simulink model "FLCS"  (Simulink 6.0)
settings: Solver=FixedStepDiscrete  StartTime=0.0  StopTime=2  RelTol=1e-3
libraries: simulink x9
settings Model: Creator=valery  LastModifiedBy=root  ExtModeAutoUpdateStatusClock=off  ProdHWDeviceType=Motorola PowerPC
settings OptimizationCC: OptimizeModelRefInitCode=on  LifeSpan=1
settings HardwareCC: ProdEndianess=BigEndian  ProdHWDeviceType=Motorola PowerPC
settings RTWCC: SystemTargetFile=mpc555rt.tlc  TemplateMakefile=mpc555rt.tmf  Description=Embedded Target for Motorola MPC555 (real-time target)  ProcessScript=mpc555rt_make_rtw_hook
settings CodeAppCC: IgnoreCustomStorageClasses=off
settings STFCustomTargetCC: TargetFcnLib=diab_tfl_tmw.mat  GenFloatMathFcnCalls=ISO_C  ModelReferenceCompliant=off  CombineOutputUpdateFcns=on  ERTCustomFileBanners=on  SystemTargetFile=mpc555rt.tlc
settings ERTTargetCC: TargetFcnLib=diab_tfl_tmw.mat  GenFloatMathFcnCalls=ISO_C  ModelReferenceCompliant=off  SupportContinuousTime=on  SupportNonInlinedSFcns=on  InlinedParameterPlacement=NonHierarchical  RootIOFormat=Individual Arguments  ERTCustomFileTemplate=example_file_process.tlc  InitialValueSource=Model
settings CustomProperty: DataType=RTWOptions_EnumType__toolbox_rtw_targets_mpc555dk_mpc555dk_mpc555rt_MPC555_OPTIMIZATION_SWITCH  Value=speed
settings EnumStrPairs: String=speed

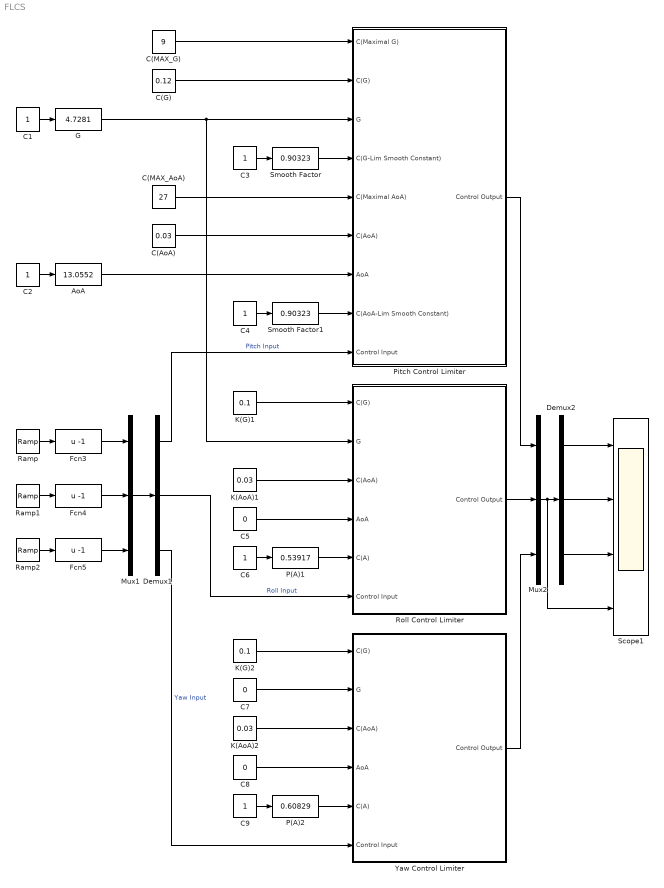
== system FLCS ==
  AoA : simulink/Math Operations/Slider Gain  low=1  gain=13.0552  high=25
  C(AoA) : Constant  Value=0.03
  C(G) : Constant  Value=0.12
  C(MAX_AoA) : Constant  Value=27
  C(MAX_G) : Constant  Value=9
  C{1..4,6,9} (6 alike) : Constant
  C5 : Constant  Value=0
  C7 : Constant  Value=0
  C8 : Constant  Value=0
  Demux1 : Demux  Outputs=3
  Demux2 : Demux  Outputs=3
  Fcn3 : Fcn  Expr=u -1
  Fcn4 : Fcn  Expr=u -1
  Fcn5 : Fcn  Expr=u -1
  G : simulink/Math Operations/Slider Gain  low=0  gain=4.7281  high=9
  K(AoA)1 : Constant  Value=0.03
  K(AoA)2 : Constant  Value=0.03
  K(G)1 : Constant  Value=0.1
  K(G)2 : Constant  Value=0.1
  Mux1 : Mux  Inputs=3
  Mux2 : Mux  Inputs=3
  P(A)1 : simulink/Math Operations/Slider Gain  low=0  gain=0.53917  high=1
  P(A)2 : simulink/Math Operations/Slider Gain  low=0  gain=0.60829  high=1
  Pitch Control Limiter : Subsystem
  Ramp : simulink/Sources/Ramp  slope=1  start=0  X0=0
  Ramp1 : simulink/Sources/Ramp  slope=1  start=0  X0=0
  Ramp2 : simulink/Sources/Ramp  slope=1  start=0  X0=0
  Roll Control Limiter : Subsystem
  Scope1 : Scope  NumInputPorts=4
      settings: YMin=-1.2~-1.2~-1.2~-1.1  YMax=1.2~1.2~1.2~1.1
  Smooth Factor : simulink/Math Operations/Slider Gain  low=0  gain=0.90323  high=1
  Smooth Factor1 : simulink/Math Operations/Slider Gain  low=0  gain=0.90323  high=1
  Yaw Control Limiter : Subsystem
  wires:
  Ramp/1 -> Fcn3/1
  Ramp1/1 -> Fcn4/1
  Ramp2/1 -> Fcn5/1
  Mux1/1 -> Demux1/1
  Fcn3/1 -> Mux1/1
  Fcn4/1 -> Mux1/2
  Fcn5/1 -> Mux1/3
  C1/1 -> G/1
  G/1 -> Pitch Control Limiter/3(G), Roll Control Limiter/2(G)
  C2/1 -> AoA/1
  C(G)/1 -> Pitch Control Limiter/2(C(G))
  Mux2/1 -> Demux2/1, Scope1/4
  Demux2/3 -> Scope1/3
  Demux2/2 -> Scope1/2
  Demux2/1 -> Scope1/1
  Demux1/1 -> Pitch Control Limiter/9(Control Input)  "Pitch Input"
  Pitch Control Limiter/1(Control Output) -> Mux2/1
  C3/1 -> Smooth Factor/1
  Smooth Factor/1 -> Pitch Control Limiter/4(C(G-Lim Smooth Constant))
  K(G)1/1 -> Roll Control Limiter/1(C(G))
  K(AoA)1/1 -> Roll Control Limiter/3(C(AoA))
  C6/1 -> P(A)1/1
  P(A)1/1 -> Roll Control Limiter/5(C(A))
  Roll Control Limiter/1(Control Output) -> Mux2/2
  Demux1/2 -> Roll Control Limiter/6(Control Input)  "Roll Input"
  C7/1 -> Yaw Control Limiter/2(G)
  C8/1 -> Yaw Control Limiter/4(AoA)
  K(G)2/1 -> Yaw Control Limiter/1(C(G))
  K(AoA)2/1 -> Yaw Control Limiter/3(C(AoA))
  C9/1 -> P(A)2/1
  P(A)2/1 -> Yaw Control Limiter/5(C(A))
  Yaw Control Limiter/1(Control Output) -> Mux2/3
  Demux1/3 -> Yaw Control Limiter/6(Control Input)  "Yaw Input"
  C5/1 -> Roll Control Limiter/4(AoA)
  C(MAX_G)/1 -> Pitch Control Limiter/1("C(Maximal G) ")
  AoA/1 -> Pitch Control Limiter/7(AoA)
  C4/1 -> Smooth Factor1/1
  Smooth Factor1/1 -> Pitch Control Limiter/8(C(AoA-Lim Smooth Constant))
  C(AoA)/1 -> Pitch Control Limiter/6(C(AoA))
  C(MAX_AoA)/1 -> Pitch Control Limiter/5(C(Maximal AoA))

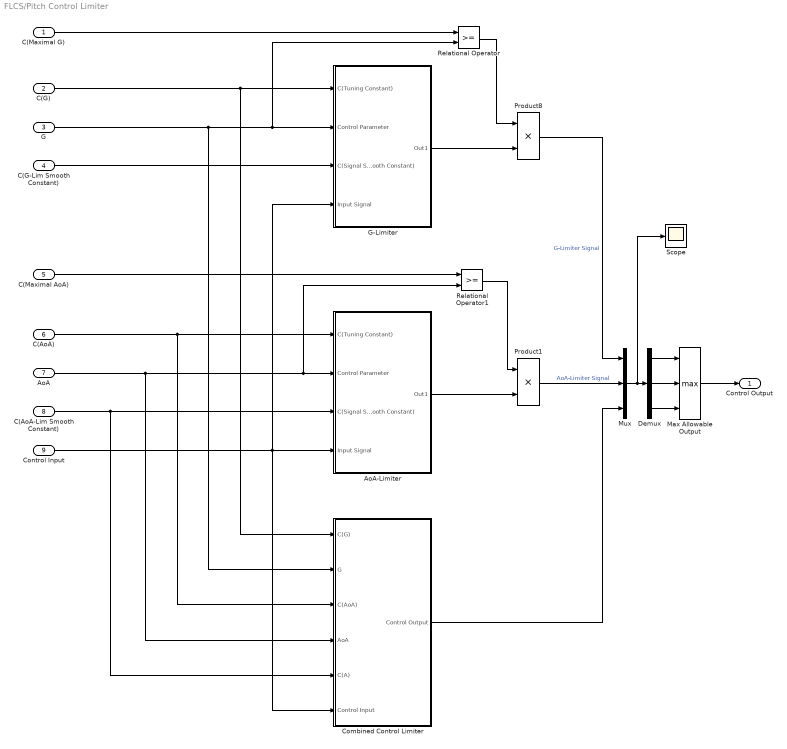
== system FLCS/Pitch Control Limiter ==
  "C(Maximal G) " : Inport  Port=1  LatchInput=off
  C(G) : Inport  Port=2  LatchInput=off
  G : Inport  Port=3  LatchInput=off
  C(G-Lim Smooth Constant) : Inport  Port=4  LatchInput=off
  C(Maximal AoA) : Inport  Port=5  LatchInput=off
  C(AoA) : Inport  Port=6  LatchInput=off
  AoA : Inport  Port=7  LatchInput=off
  C(AoA-Lim Smooth Constant) : Inport  Port=8  LatchInput=off
  Control Input : Inport  Port=9  LatchInput=off
  AoA-Limiter : Subsystem
  Combined Control Limiter : Subsystem
  Demux : Demux  Outputs=3
  G-Limiter : Subsystem
  Max Allowable Output : MinMax  Function=max  Inputs=3
  Mux : Mux  Inputs=3
  Product1 : Product  RndMeth=Zero
  Product8 : Product  RndMeth=Zero
  Relational Operator : RelationalOperator  LogicOutDataTypeMode=Boolean
  Relational Operator1 : RelationalOperator  LogicOutDataTypeMode=Boolean
  Scope : Scope
      settings: YMin=-1.1  YMax=1.1
  Control Output : Outport
  wires:
  "C(Maximal G) "/1 -> Relational Operator/1
  Relational Operator/1 -> Product8/1
  G-Limiter/1(Out1) -> Product8/2
  C(G)/1 -> G-Limiter/1(C(Tuning Constant)), Combined Control Limiter/1(C(G))
  G/1 -> G-Limiter/2(Control Parameter), Relational Operator/2, Combined Control Limiter/2(G)
  C(G-Lim Smooth Constant)/1 -> G-Limiter/3(C(Signal Smooth Constant))
  C(AoA)/1 -> AoA-Limiter/1(C(Tuning Constant)), Combined Control Limiter/3(C(AoA))
  C(AoA-Lim Smooth Constant)/1 -> AoA-Limiter/3(C(Signal Smooth Constant)), Combined Control Limiter/5(C(A))
  C(Maximal AoA)/1 -> Relational Operator1/1
  Relational Operator1/1 -> Product1/1
  AoA-Limiter/1(Out1) -> Product1/2
  Control Input/1 -> AoA-Limiter/4(Input Signal), G-Limiter/4(Input Signal), Combined Control Limiter/6(Control Input)
  Max Allowable Output/1 -> Control Output/1
  Product1/1 -> Mux/2  "AoA-Limiter Signal"
  Product8/1 -> Mux/1  "G-Limiter Signal"
  Combined Control Limiter/1(Control Output) -> Mux/3
  AoA/1 -> AoA-Limiter/2(Control Parameter), Relational Operator1/2, Combined Control Limiter/4(AoA)
  Mux/1 -> Demux/1, Scope/1
  Demux/1 -> Max Allowable Output/1
  Demux/2 -> Max Allowable Output/2
  Demux/3 -> Max Allowable Output/3

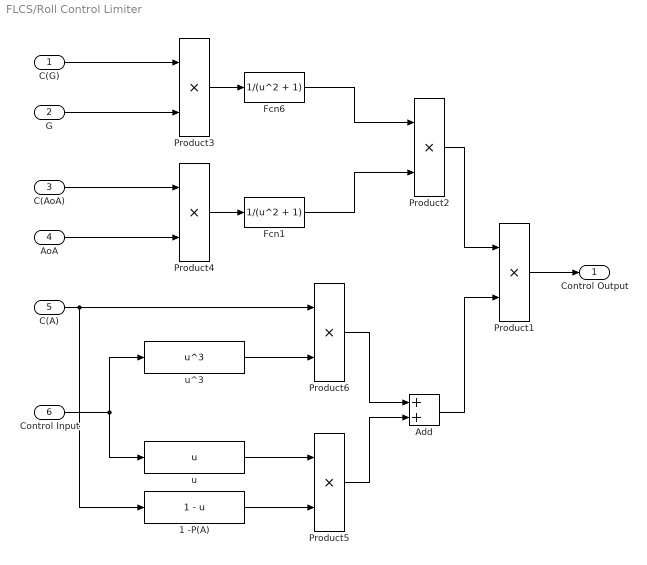
== system FLCS/Roll Control Limiter ==
  C(G) : Inport  Port=1  LatchInput=off
  G : Inport  Port=2  LatchInput=off
  C(AoA) : Inport  Port=3  LatchInput=off
  AoA : Inport  Port=4  LatchInput=off
  C(A) : Inport  Port=5  LatchInput=off
  Control Input : Inport  Port=6  LatchInput=off
  1 -P(A) : Fcn  Expr=1 - u
  Add : Sum  OutScaling=2^-10
  Fcn1 : Fcn  Expr=1/(u^2 + 1)
  Fcn6 : Fcn  Expr=1/(u^2 + 1)
  Product{1..6} (6 alike) : Product  RndMeth=Zero
  u : Fcn  Expr=u
  u^3 : Fcn  Expr=u^3
  Control Output : Outport
  wires:
  Product1/1 -> Control Output/1
  Control Input/1 -> u^3/1, u/1
  C(G)/1 -> Product3/1
  Product3/1 -> Fcn6/1
  Product4/1 -> Fcn1/1
  C(A)/1 -> 1 -P(A)/1, Product6/1
  u^3/1 -> Product6/2
  Product6/1 -> Add/1
  Product5/1 -> Add/2
  u/1 -> Product5/1
  1 -P(A)/1 -> Product5/2
  C(AoA)/1 -> Product4/1
  AoA/1 -> Product4/2
  G/1 -> Product3/2
  Fcn6/1 -> Product2/1
  Fcn1/1 -> Product2/2
  Add/1 -> Product1/2
  Product2/1 -> Product1/1

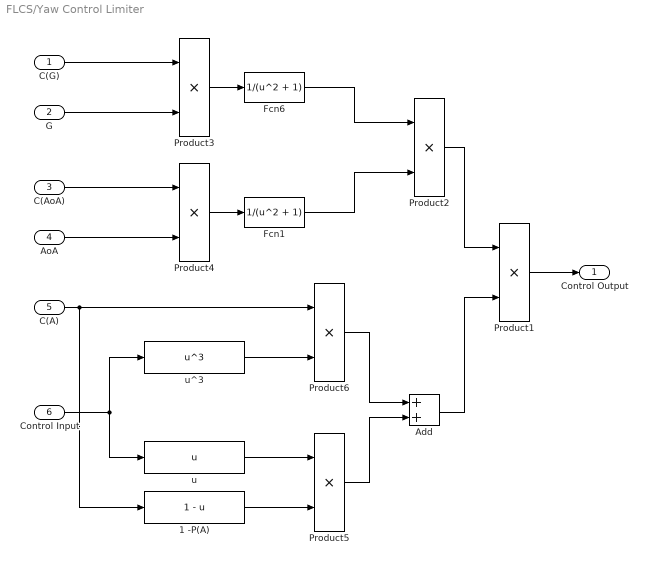
== system FLCS/Yaw Control Limiter ==
  C(G) : Inport  Port=1  LatchInput=off
  G : Inport  Port=2  LatchInput=off
  C(AoA) : Inport  Port=3  LatchInput=off
  AoA : Inport  Port=4  LatchInput=off
  C(A) : Inport  Port=5  LatchInput=off
  Control Input : Inport  Port=6  LatchInput=off
  1 -P(A) : Fcn  Expr=1 - u
  Add : Sum  OutScaling=2^-10
  Fcn1 : Fcn  Expr=1/(u^2 + 1)
  Fcn6 : Fcn  Expr=1/(u^2 + 1)
  Product{1..6} (6 alike) : Product  RndMeth=Zero
  u : Fcn  Expr=u
  u^3 : Fcn  Expr=u^3
  Control Output : Outport
  wires:
  Product1/1 -> Control Output/1
  Control Input/1 -> u^3/1, u/1
  C(G)/1 -> Product3/1
  Product3/1 -> Fcn6/1
  Product4/1 -> Fcn1/1
  C(A)/1 -> 1 -P(A)/1, Product6/1
  u^3/1 -> Product6/2
  Product6/1 -> Add/1
  Product5/1 -> Add/2
  u/1 -> Product5/1
  1 -P(A)/1 -> Product5/2
  C(AoA)/1 -> Product4/1
  AoA/1 -> Product4/2
  G/1 -> Product3/2
  Fcn6/1 -> Product2/1
  Fcn1/1 -> Product2/2
  Add/1 -> Product1/2
  Product2/1 -> Product1/1

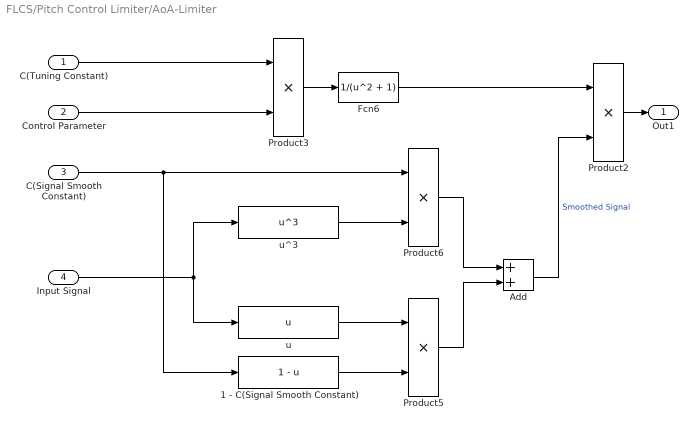
== system FLCS/Pitch Control Limiter/AoA-Limiter ==
  C(Tuning Constant) : Inport  Port=1  LatchInput=off
  Control Parameter : Inport  Port=2  LatchInput=off
  C(Signal Smooth Constant) : Inport  Port=3  LatchInput=off
  Input Signal : Inport  Port=4  LatchInput=off
  1 - C(Signal Smooth Constant) : Fcn  Expr=1 - u
  Add : Sum  OutScaling=2^-10
  Fcn6 : Fcn  Expr=1/(u^2 + 1)
  Product{2..3,5..6} (4 alike) : Product  RndMeth=Zero
  u : Fcn  Expr=u
  u^3 : Fcn  Expr=u^3
  Out1 : Outport
  wires:
  Input Signal/1 -> u/1, u^3/1
  C(Tuning Constant)/1 -> Product3/1
  Product3/1 -> Fcn6/1
  C(Signal Smooth Constant)/1 -> Product6/1, 1 - C(Signal Smooth Constant)/1
  u^3/1 -> Product6/2
  Product6/1 -> Add/1
  Product5/1 -> Add/2
  u/1 -> Product5/1
  1 - C(Signal Smooth Constant)/1 -> Product5/2
  Control Parameter/1 -> Product3/2
  Fcn6/1 -> Product2/1
  Add/1 -> Product2/2  "Smoothed Signal"
  Product2/1 -> Out1/1

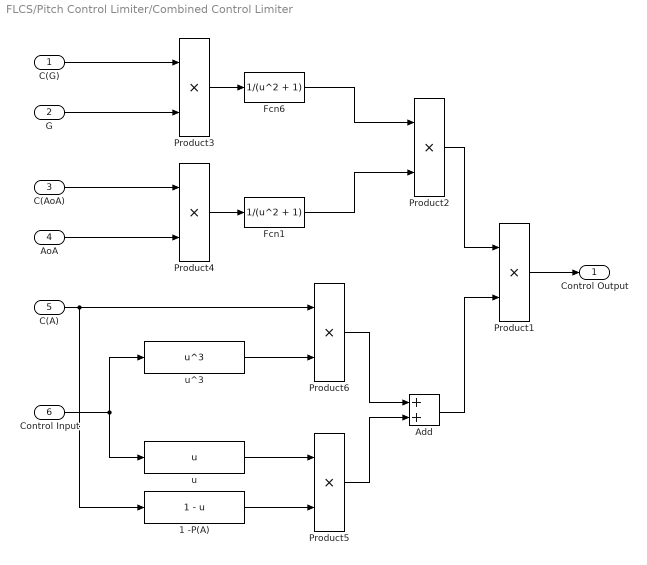
== system FLCS/Pitch Control Limiter/Combined Control Limiter ==
  C(G) : Inport  Port=1  LatchInput=off
  G : Inport  Port=2  LatchInput=off
  C(AoA) : Inport  Port=3  LatchInput=off
  AoA : Inport  Port=4  LatchInput=off
  C(A) : Inport  Port=5  LatchInput=off
  Control Input : Inport  Port=6  LatchInput=off
  1 -P(A) : Fcn  Expr=1 - u
  Add : Sum  OutScaling=2^-10
  Fcn1 : Fcn  Expr=1/(u^2 + 1)
  Fcn6 : Fcn  Expr=1/(u^2 + 1)
  Product{1..6} (6 alike) : Product  RndMeth=Zero
  u : Fcn  Expr=u
  u^3 : Fcn  Expr=u^3
  Control Output : Outport
  wires:
  Product1/1 -> Control Output/1
  Control Input/1 -> u^3/1, u/1
  C(G)/1 -> Product3/1
  Product3/1 -> Fcn6/1
  Product4/1 -> Fcn1/1
  C(A)/1 -> 1 -P(A)/1, Product6/1
  u^3/1 -> Product6/2
  Product6/1 -> Add/1
  Product5/1 -> Add/2
  u/1 -> Product5/1
  1 -P(A)/1 -> Product5/2
  C(AoA)/1 -> Product4/1
  AoA/1 -> Product4/2
  G/1 -> Product3/2
  Fcn6/1 -> Product2/1
  Fcn1/1 -> Product2/2
  Add/1 -> Product1/2
  Product2/1 -> Product1/1

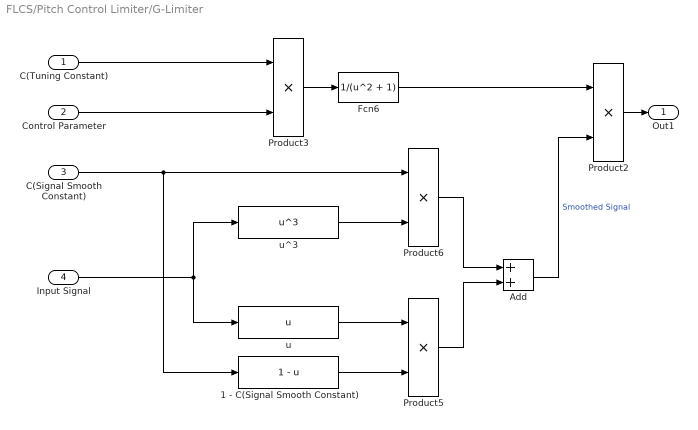
== system FLCS/Pitch Control Limiter/G-Limiter ==
  C(Tuning Constant) : Inport  Port=1  LatchInput=off
  Control Parameter : Inport  Port=2  LatchInput=off
  C(Signal Smooth Constant) : Inport  Port=3  LatchInput=off
  Input Signal : Inport  Port=4  LatchInput=off
  1 - C(Signal Smooth Constant) : Fcn  Expr=1 - u
  Add : Sum  OutScaling=2^-10
  Fcn6 : Fcn  Expr=1/(u^2 + 1)
  Product{2..3,5..6} (4 alike) : Product  RndMeth=Zero
  u : Fcn  Expr=u
  u^3 : Fcn  Expr=u^3
  Out1 : Outport
  wires:
  Input Signal/1 -> u/1, u^3/1
  C(Tuning Constant)/1 -> Product3/1
  Product3/1 -> Fcn6/1
  C(Signal Smooth Constant)/1 -> Product6/1, 1 - C(Signal Smooth Constant)/1
  u^3/1 -> Product6/2
  Product6/1 -> Add/1
  Product5/1 -> Add/2
  u/1 -> Product5/1
  1 - C(Signal Smooth Constant)/1 -> Product5/2
  Control Parameter/1 -> Product3/2
  Fcn6/1 -> Product2/1
  Add/1 -> Product2/2  "Smoothed Signal"
  Product2/1 -> Out1/1
